simulink model "non_linear"  (R2020a)
settings: Solver=VariableStepAuto  StartTime=0.0  StopTime=10.0  RelTol=1e-3
values from neighbouring files (symbols this model uses):
  G = 9.8    [main.m]
  Kt = 3.575e-5    (= 3.575e-05)    [main.m]
  M = 1    [main.m]
  omega_0 = sqrt(G*M/Kt)    [main.m]
  u_0 = omega_0    [main.m]
  Z0 = 2    [main.m]
settings Model: Creator=josem  LastModifiedBy=josem

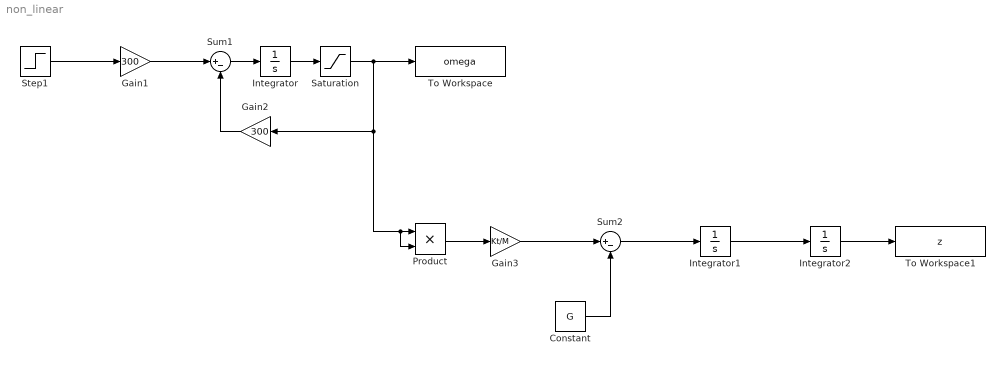
== system non_linear ==
  Constant : Constant  Value=G
  Gain1 : Gain  Gain=300
  Gain2 : Gain  Gain=300
  Gain3 : Gain  Gain=Kt/M
  Integrator : Integrator  InitialCondition=omega_0
  Integrator1 : Integrator
  Integrator2 : Integrator  InitialCondition=Z0
  Product : Product
  Saturation : Saturate  UpperLimit=3*omega_0  LowerLimit=0
  Step1 : Step  Before=u_0  After=u  SampleTime=0
  Sum1 : Sum  Inputs=|+-
  Sum2 : Sum  Inputs=|+-
  To Workspace : ToWorkspace  VariableName=omega  SaveFormat=Structure With Time  SampleTime=-1
  To Workspace1 : ToWorkspace  VariableName=z  SaveFormat=Structure With Time  SampleTime=-1
  wires:
  Integrator/1 -> Saturation/1
  Step1/1 -> Gain1/1
  Gain1/1 -> Sum1/1
  Sum1/1 -> Integrator/1
  Gain2/1 -> Sum1/2
  Product/1 -> Gain3/1
  Gain3/1 -> Sum2/1
  Constant/1 -> Sum2/2
  Sum2/1 -> Integrator1/1
  Integrator1/1 -> Integrator2/1
  Integrator2/1 -> To Workspace1/1
  Saturation/1 -> Product/2, Product/1, Gain2/1, To Workspace/1
